simulink library "CurrentsLib"  (Simulink 7.7)
settings: Solver=ode45  SolverMode=SingleTasking  StartTime=0.0  StopTime=10.0  RelTol=1e-3
undefined symbols (not defined in the file or in its folder): A, B, diff1, EX, G, gX, PfAHP, PmAHP, PsAHP, Q0, S, T
libraries: CurrentsLib x75, WaveformsLib x11
(part 1 of 2)
settings Model: Creator=jpalma  LastModifiedBy=jpalma

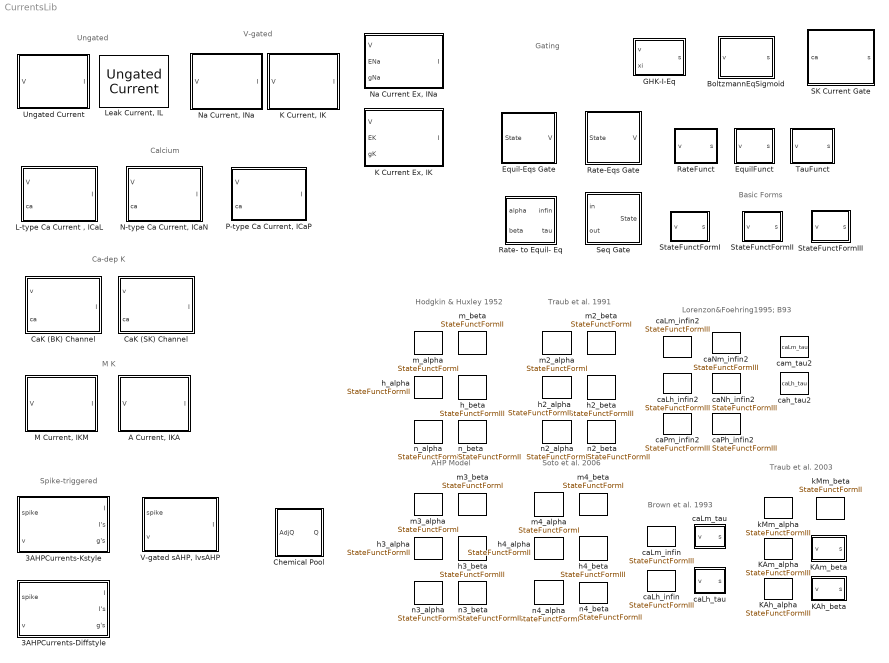
== system CurrentsLib ==
  note: Hodgkin & Huxley 1952
  note: Soto et al. 2006
  note: Basic Forms
  note: Traub et al. 1991
  note: AHP Model
  note: Gating
  note: V-gated
  note: Ungated
  note: Spike-triggered
  note: Brown et al. 1993
  note: Lorenzon&Foehring1995; B93
  note: Calcium
  note: Ca-dep K
  note: Traub et al. 2003
  note: M K
  3AHPCurrents-Diffstyle : Subsystem  mask{EfAHP=PfAHP(1), gfAHP=PfAHP(2), tauRfAHP=PfAHP(3), tauFfAHP=PfAHP(4), EmAHP=PmAHP(1), gmAHP=PmAHP(2), tauRmAHP=PmAHP(3), tauFmAHP=PmAHP(4), EsAHP=PsAHP(1), gsAHP=PsAHP(2), tauRsAHP=PsAHP(3), tauFsAHP=PsAHP(4)}
      mask prompts: EfAHP "Eq fAHP, EfAHP"; gfAHP "Conductance fAHP, gfAHP"; tauRfAHP "Rise Time fAHP"; tauFfAHP "Fall Time fAHP"; EmAHP "Eq mAHP, EmAHP"; gmAHP "Conductance mAHP, gmAHP"; tauRmAHP "Rise Time mAHP"; tauFmAHP "Fall Time mAHP"; EsAHP "Eq sAHP, EsAHP"; gsAHP "Conductance sAHP, gsAHP"; tauRsAHP "Rise Time sAHP"; tauFsAHP "Fall Time sAHP"
      mask help: Author: Jesse Palma
      mask Help: Author: Jesse Palma
      mask TabNameString: fAHP,fAHP,fAHP,fAHP,mAHP,mAHP,mAHP,mAHP,sAHP,sAHP,sAHP,sAHP
      mask Display: image(imread('../Libs/icons/ChannelV.jpg'),'center');
  3AHPCurrents-Kstyle : Subsystem  mask{EfAHP=PfAHP(1), gfAHP=PfAHP(2), tauRfAHP=PfAHP(3), tauFfAHP=PfAHP(4), EmAHP=PmAHP(1), gmAHP=PmAHP(2), tauRmAHP=PmAHP(3), tauFmAHP=PmAHP(4), EsAHP=PsAHP(1), gsAHP=PsAHP(2), tauRsAHP=PsAHP(3), tauFsAHP=PsAHP(4)}
      mask prompts: EfAHP "Eq fAHP, EfAHP"; gfAHP "Conductance fAHP, gfAHP"; tauRfAHP "Rise Time fAHP"; tauFfAHP "Fall Time fAHP"; EmAHP "Eq mAHP, EmAHP"; gmAHP "Conductance mAHP, gmAHP"; tauRmAHP "Rise Time mAHP"; tauFmAHP "Fall Time mAHP"; EsAHP "Eq sAHP, EsAHP"; gsAHP "Conductance sAHP, gsAHP"; tauRsAHP "Rise Time sAHP"; tauFsAHP "Fall Time sAHP"
      mask help: Author: Jesse Palma
      mask Help: Author: Jesse Palma
      mask TabNameString: fAHP,fAHP,fAHP,fAHP,mAHP,mAHP,mAHP,mAHP,sAHP,sAHP,sAHP,sAHP
      mask Display: image(imread('../Libs/icons/ChannelV.jpg'),'center');
  "A Current, IKA" : Subsystem  mask{EKA=-70, gKA=0.1, m_a=KAm_alpha, m_b=KAm_beta, h_a=KAh_alpha, h_b=KAh_beta}
      mask prompts: EKA "A Equilibrium, EKA (mV)"; gKA "A Conductance, gKA (mS/cm^2)"; m_a "Activation m Fwd Rate Eq, m_a"; m_b "Activation m Bckwd Rate Eq, m_b"; h_a "Inactivation h Fwd Rate Eq, h_a"; h_b "Inactivation h Bckwd Rate Eq, h_b"
      mask help:
      | Potassium A Current
      | IKA =  gKA m^4 h (EKA - V)
      |
      | (Traub et al. 2003)
      mask init:
      | set_param([gcb '/m Rate-Eqs Gate'], 'alphaF', m_a);
      | set_param([gcb '/m Rate-Eqs Gate'], 'betaF', m_b);
      | set_param([gcb '/h Rate-Eqs Gate'], 'alphaF', h_a);
      | set_param([gcb '/h Rate-Eqs Gate'], 'betaF', h_b);
      mask Help:
      | Potassium A Current
      | IKA =  gKA m^4 h (EKA - V)
      | 
      | (Traub et al. 2003)
      mask StyleString: edit,edit,popup(KAm_alpha),popup(KAm_beta),popup(KAh_alpha),popup(KAh_beta)
      mask TabNameString: Basic,Basic,Gating,Gating,Gating,Gating
      mask Display: image(imread('../Libs/icons/ChannelV.jpg'),'center');
  BoltzmannEqSigmoid : Subsystem  mask{v05=-20, k=1/5, g=4}
      mask prompts: v05 "Inflexion Point, v_0.5"; k "Slope factor, k"; g "Gain, g"
      mask help:
      | Boltzmann Equation as Sigmoid with Gain
      | [See (Dobois et al., 2009), doi:10.1016/j.pbiomolbio.2009.07.001]
      |
      |    s = g / (1 + exp((v_0.5-v)/k)
      |
      |    where k = zF/RT (slope factor)
      mask Help:
      | Boltzmann Equation as Sigmoid with Gain
      | [See (Dobois et al., 2009), doi:10.1016/j.pbiomolbio.2009.07.001]
      | 
      |    s = g / (1 + exp((v_0.5-v)/k))
      | 
      |    where k = zF/RT (Slope factor)
      mask Display: image(imread('../Libs/icons/SigmoidSF.jpg'),'center');
  CaK (BK) Channel : Subsystem  mask{EBK=-65, gBK=4.0}
      mask Display: image(imread('../Libs/icons/ChannelVC.jpg'),'center');
  CaK (SK) Channel : Subsystem  mask{ESK=-100, gSK=0.5}
      mask prompts: ESK "SK Equilibrium Potential, ESK"; gSK "SK Conductance, gSK"
      mask Display: image(imread('../Libs/icons/ChannelVC.jpg'),'center');
  Chemical Pool : Subsystem  mask{f=10/(69843), d=1/1000, a=1/200}
  Equil-Eqs Gate : Subsystem  mask{equilF=caLh_infin, tauF=caLh_tau}
      mask prompts: equilF "Equilbrium Eq (Steady State)"; tauF "Tau Eq (Time constant)"
      mask help: dF/dt = ( infty_F-F) / tau_F
      mask init:
      | set_param([gcb '/TauFunct'], 'BlockChoice', tauF);
      | set_param([gcb '/EquilFunct'], 'BlockChoice', equilF);
      mask Help: dF/dt = ( infty_F-F) / tau_F
      mask StyleString: popup(caLm_infin|caLh_infin|caLm_infin2|caLh_infin2|caNm_infin2|caNh_infin2|caPm_infin2|caPh_infin2),popup(caLm_tau|caLh_tau|cam_tau2|cah_tau2)
      mask Display: image(imread('../Libs/icons/EquilEq.jpg'),'center');
  EquilFunct : Subsystem  BlockChoice=caLh_infin
      settings: TemplateBlock=self  MemberBlocks=caLh_infin,caLh_infin2,caLm_infin,caLm_infin2,caNh_infin2,caNm_infin2,caPh_infin2,caPm_infin2
  GHK-I-Eq : Subsystem  mask{z=2, Xi=10*10^(-6), Xo=5, P=3.4*10^(-5)}
      mask prompts: z "Ion charge, z"; Xi "Internal concentration, Xi"; Xo "External concentration, Xo"; P "Permeability Scaling Factor, P"
      mask help:
      | GHK Current Equation
      |
      |    s = {PFz} kV (Xi-Xo exp (-kV))/(1 - exp(-kV))
      |
      |    where k = zF/RT
      |
      | {PFz} is a scaling factor, based on permeability
      |
      | z is the valence of ion
      | V is the transmembrane potential in volts
      | F is the Faraday constant, equal to 96,485 C·mol-1 or J·V-1·mol-1
      | R is the gas constant, equal to 8.314 J·K-1·mol-1
      | T is the absolute temperature, measured in kelvins (= degrees Celsius + 273.15)
      | Xi is the intracellular concentration of ion, measured in mol·m-3 or mmol·l-1
      | Xo is the extracellular concentration of ion, measured in mol·m-3
      mask Help:
      | GHK Current Equation
      | 
      |    s = {PFz} kV (Xi-Xo exp (-kV))/(1 - exp(-kV))
      | 
      |    where k = zF/RT
      | 
      | {PFz} is removed because it is scaling factor, which is performed outside this block
      | 
      | z is the valence of ion
      | V is the transmembrane potential in volts
      | F is the Faraday constant, equal to 96,485 C·mol-1 or J·V-1·mol-1
      | R is the gas constant, equal to 8.314 J·K-1·mol-1
      | T is the absolute temperature, measured in kelvins (= degrees Celsius + 273.15)
      | Xi is the intracellular concentration of ion, measured in mol·m-3 or mmol·l-1
      | Xo is the extracellular concentration of ion, measured in mol·m-3
  "K Current Ex, IK" : Subsystem  mask{n_a=n3_alpha, n_b=n3_beta}
      mask prompts: n_a "Activation n Fwd Rate Eq, n_a"; n_b "Activation n Bckwd Rate Eq, n_b"
      mask help:
      | Basic Potassium Current (Delayed Rectifier)
      |  IK =  gK n^4 (EK - V)
      |
      |  Model 1: Hodgkin & Huxley
      |  Model 2: Traub et al. 1991
      |  Model 3: AHP Model
      |           EK=-100 mV, gK = 16 mS/cm^2
      |  Model 4: Soto et al. 2006
      mask init:
      | set_param([gcb '/n Rate-Eqs Gate'], 'alphaF', n_a);
      | set_param([gcb '/n Rate-Eqs Gate'], 'betaF', n_b);
      mask Help:
      | Basic Potassium Current (Delayed Rectifier)
      |  IK =  gK n^4 (EK - V)
      | 
      |  Model 1: Hodgkin & Huxley
      |  Model 2: Traub et al. 1991
      |  Model 3: AHP Model
      |           EK=-100 mV, gK = 16 mS/cm^2
      |  Model 4: Soto et al. 2006
      mask StyleString: popup(n_alpha|n2_alpha|n3_alpha|n4_alpha),popup(n_beta|n2_beta|n3_beta|n4_beta)
      mask TabNameString: Gating,Gating
      mask Display: image(imread('../Libs/icons/ChannelV.jpg'),'center');
  "K Current, IK" : Subsystem  mask{EK=-100, gK=16, n_a=n3_alpha, n_b=n3_beta}
      mask prompts: EK "Potassium Equilibrium, EK (mV)"; gK "Potassium Conductance, gK (mS/cm^2)"; n_a "Activation n Fwd Rate Eq, n_a"; n_b "Activation n Bckwd Rate Eq, n_b"
      mask help:
      | Basic Potassium Current (Delayed Rectifier)
      |  IK =  gK n^4 (EK - V)
      |
      |  Model 1: Hodgkin & Huxley
      |  Model 2: Traub et al. 1991
      |  Model 3: AHP Model
      |           EK=-100 mV, gK = 16 mS/cm^2
      |  Model 4: Soto et al. 2006
      mask init:
      | set_param([gcb '/n Rate-Eqs Gate'], 'alphaF', n_a);
      | set_param([gcb '/n Rate-Eqs Gate'], 'betaF', n_b);
      mask Help:
      | Basic Potassium Current (Delayed Rectifier)
      |  IK =  gK n^4 (EK - V)
      | 
      |  Model 1: Hodgkin & Huxley
      |  Model 2: Traub et al. 1991
      |  Model 3: AHP Model
      |           EK=-100 mV, gK = 16 mS/cm^2
      |  Model 4: Soto et al. 2006
      mask StyleString: edit,edit,popup(n_alpha|n2_alpha|n3_alpha|n4_alpha),popup(n_beta|n2_beta|n3_beta|n4_beta)
      mask TabNameString: Basic,Basic,Gating,Gating
      mask Display: image(imread('../Libs/icons/ChannelV.jpg'),'center');
  KAh_alpha : CurrentsLib/StateFunctFormIII  SystemSampleTime=-1  T=-85  S=-1/16  B=1  G=1/8
  KAh_beta : Subsystem
      mask Description: 1.2
      mask Help: 1.2
  KAm_alpha : CurrentsLib/StateFunctFormIII  SystemSampleTime=-1  T=-28  S=1/22.5  B=1  G=1/8
  KAm_beta : Subsystem
  "L-type Ca Current , ICaL" : Subsystem  mask{ECaL=130, gCaL=0.1, m_e=caLm_infin2, m_t=cam_tau2, h_e=caLh_infin2, h_t=cah_tau2}
      mask prompts: ECaL "Sodium Equilibrium, ECaL (mV)"; gCaL "Sodium Conductance, gCaL (mS/cm^2)"; m_e "Activation m Equil Eq, m_e"; m_t "Activation m Tau Eq, m_t"; h_e "Inactivation h Equil Eq, h_e"; h_t "Inactivation h Tau Eq, h_t"
      mask help:
      | L-type Calcium Current
      | ICaL =  gCaL m^2 h (ECaL - V)
      |
      | Based on (Brown et al. 1993)
      mask init:
      | set_param([gcb '/m Equil-Eqs Gate'], 'equilF', m_e);
      | set_param([gcb '/m Equil-Eqs Gate'], 'tauF', m_t);
      | set_param([gcb '/h Equil-Eqs Gate'], 'equilF', h_e);
      | set_param([gcb '/h Equil-Eqs Gate'], 'tauF', h_t);
      mask Help:
      | L-type Calcium Current
      | ICaL =  gCaL m^2 h (ECaL - V)
      | 
      | Based on (Brown et al. 1993)
      mask StyleString: edit,edit,popup(caLm_infin|caLm_infin2),popup(caLm_tau|cam_tau2),popup(caLh_infin|caLh_infin2),popup(caLh_tau|cah_tau2)
      mask TabNameString: Basic,Basic,Gating,Gating,Gating,Gating
      mask Display: image(imread('../Libs/icons/ChannelV.jpg'),'center');
  "Leak Current, IL" : CurrentsLib/Ungated Current  SystemSampleTime=-1  EX=-65  gX=0.1
  "M Current, IKM" : Subsystem  mask{EK=-100, gK=0.1, m_a=kMm_alpha, m_b=kMm_beta}
      mask prompts: EK "Potassium Equilibrium, EK (mV)"; gK "Potassium Conductance, gK (mS/cm^2)"; m_a "Activation m Fwd Rate Eq, m_a"; m_b "Activation m Bckwd Rate Eq, m_b"
      mask help: Potassium M Current (Traub et al. 2003)
      mask init:
      | set_param([gcb '/m Rate-Eqs Gate'], 'alphaF', m_a);
      | set_param([gcb '/m Rate-Eqs Gate'], 'betaF', m_b);
      mask Help: Potassium M Current (Traub et al. 2003)
      mask StyleString: edit,edit,popup(kMm_alpha),popup(kMm_beta)
      mask TabNameString: Basic,Basic,Gating,Gating
      mask Display: image(imread('../Libs/icons/ChannelV.jpg'),'center');
  "N-type Ca Current, ICaN" : Subsystem  mask{ECaN=130, gCaN=0.1, m_e=caNm_infin2, m_t=cam_tau2, h_e=caNh_infin2, h_t=cah_tau2}
      mask prompts: ECaN "Sodium Equilibrium, ECaN (mV)"; gCaN "Sodium Conductance, gCaN (mS/cm^2)"; m_e "Activation m Equil Eq, m_e"; m_t "Activation m Tau Eq, m_t"; h_e "Inactivation h Equil Eq, h_e"; h_t "Inactivation h Tau Eq, h_t"
      mask help:
      | N-type Calcium Current
      | ICaN =  gCaN m h (ECaN - V)
      mask init: same as CurrentsLib/L-type Ca Current , ICaL
      mask Help:
      | N-type Calcium Current
      | ICaN =  gCaN m h (ECaN - V)
      mask StyleString: edit,edit,popup(caNm_infin|caNm_infin2),popup(caNm_tau|cam_tau2),popup(caNh_infin|caNh_infin2),popup(caNh_tau|cah_tau2)
      mask TabNameString: Basic,Basic,Gating,Gating,Gating,Gating
      mask Display: image(imread('../Libs/icons/ChannelV.jpg'),'center');
  "Na Current Ex, INa" : Subsystem  mask{m_a=m3_alpha, m_b=m3_beta, h_a=h3_alpha, h_b=h3_beta}
      mask prompts: m_a "Activation m Fwd Rate Eq, m_a"; m_b "Activation m Bckwd Rate Eq, m_b"; h_a "Inactivation h Fwd Rate Eq, h_a"; h_b "Inactivation h Bckwd Rate Eq, h_b"
      mask help:
      | Basic Sodium Current
      | INa =  gNa m^3 h (ENa - V)
      |
      |  Model 1: Hodgkin & Huxley
      |  Model 2: Traub et al. 1991
      |  Model 3: AHP Model
      |           ENa=50 mV, gNa = 45 mS/cm^2
      |  Model 4: Soto et al. 2006
      mask init: same as CurrentsLib/A Current, IKA
      mask Help:
      | Basic Sodium Current
      | INa =  gNa m^3 h (ENa - V)
      | 
      |  Model 1: Hodgkin & Huxley
      |  Model 2: Traub et al. 1991
      |  Model 3: AHP Model
      |           ENa=50 mV, gNa = 45 mS/cm^2
      |  Model 4: Soto et al. 2006
      mask StyleString: popup(m_alpha|m2_alpha|m3_alpha|m4_alpha),popup(m_beta|m2_beta|m3_beta|m4_beta),popup(h_alpha|h2_alpha|h3_alpha|h4_alpha),popup(h_beta|h2_beta|h3_beta|h4_beta)
      mask TabNameString: Gating,Gating,Gating,Gating
      mask Display: image(imread('../Libs/icons/ChannelV.jpg'),'center');
  "Na Current, INa" : Subsystem  mask{ENa=50, gNa=45, m_a=m3_alpha, m_b=m3_beta, h_a=h3_alpha, h_b=h3_beta}
      mask prompts: ENa "Sodium Equilibrium, ENa (mV)"; gNa "Sodium Conductance, gNa (mS/cm^2)"; m_a "Activation m Fwd Rate Eq, m_a"; m_b "Activation m Bckwd Rate Eq, m_b"; h_a "Inactivation h Fwd Rate Eq, h_a"; h_b "Inactivation h Bckwd Rate Eq, h_b"
      mask help:
      | Basic Sodium Current
      | INa =  gNa m^3 h (ENa - V)
      |
      |  Model 1: Hodgkin & Huxley
      |  Model 2: Traub et al. 1991
      |  Model 3: AHP Model
      |           ENa=50 mV, gNa = 45 mS/cm^2
      |  Model 4: Soto et al. 2006
      mask init: same as CurrentsLib/A Current, IKA
      mask Help:
      | Basic Sodium Current
      | INa =  gNa m^3 h (ENa - V)
      | 
      |  Model 1: Hodgkin & Huxley
      |  Model 2: Traub et al. 1991
      |  Model 3: AHP Model
      |           ENa=50 mV, gNa = 45 mS/cm^2
      |  Model 4: Soto et al. 2006
      mask StyleString: edit,edit,popup(m_alpha|m2_alpha|m3_alpha|m4_alpha),popup(m_beta|m2_beta|m3_beta|m4_beta),popup(h_alpha|h2_alpha|h3_alpha|h4_alpha),popup(h_beta|h2_beta|h3_beta|h4_beta)
      mask TabNameString: Basic,Basic,Gating,Gating,Gating,Gating
      mask Display: image(imread('../Libs/icons/ChannelV.jpg'),'center');
  "P-type Ca Current, ICaP" : Subsystem  mask{ECaP=130, gCaP=0.1, m_e=caPm_infin2, m_t=cam_tau2, h_e=caPh_infin2, h_t=cah_tau2}
      mask prompts: ECaP "Sodium Equilibrium, ECaP (mV)"; gCaP "Sodium Conductance, gCaP (mS/cm^2)"; m_e "Activation m Equil Eq, m_e"; m_t "Activation m Tau Eq, m_t"; h_e "Inactivation h Equil Eq, h_e"; h_t "Inactivation h Tau Eq, h_t"
      mask help:
      | P-type Calcium Current
      | ICaP =  gCaP m h (ECaP - V)
      mask init: same as CurrentsLib/L-type Ca Current , ICaL
      mask Help:
      | P-type Calcium Current
      | ICaP =  gCaP m h (ECaP - V)
      mask StyleString: edit,edit,popup(caPm_infin|caPm_infin2),popup(caPm_tau|cam_tau2),popup(caPh_infin|caPh_infin2),popup(caPh_tau|cah_tau2)
      mask TabNameString: Basic,Basic,Gating,Gating,Gating,Gating
      mask Display: image(imread('../Libs/icons/ChannelV.jpg'),'center');
  Rate- to Equil- Eq : Subsystem
      mask Description: Converts Rate Eqs to Equil Eqs
      mask Help: Converts Rate Eqs to Equil Eqs
      mask Display: image(imread('../Libs/icons/Rate2Equil.jpg'),'center');
  Rate-Eqs Gate : Subsystem  mask{alphaF=m3_alpha, betaF=m3_beta}
      mask prompts: alphaF "Forward Rate Eq"; betaF "Backward Rate Eq"
      mask help: dF/dt = alpha_F(1-F) - beta_F*F
      mask init:
      | set_param([gcb '/RateFunctA'], 'BlockChoice', alphaF);
      | set_param([gcb '/RateFunctB'], 'BlockChoice', betaF);
      mask Help: dF/dt =  alpha_F(1-F) - beta_F*F
      mask StyleString: popup(m_alpha|h_alpha|n_alpha|m2_alpha|h2_alpha|n2_alpha|m3_alpha|h3_alpha|n3_alpha|m4_alpha|h4_alpha|n4_alpha|kMm_alpha|KAm_alpha|KAh_alpha),popup(m_beta|h_beta|n_beta|m2_beta|h2_beta|n2_beta|m3_beta|h3_beta|n3_beta|m4_beta|h4_beta|n4_beta|kMm_beta|KAm_beta|KAh_beta)
      mask Display: image(imread('../Libs/icons/RateEq.jpg'),'center');
  RateFunct : Subsystem  BlockChoice=m_alpha
      settings: TemplateBlock=self  MemberBlocks=KAh_alpha,KAh_beta,KAm_alpha,KAm_beta,caLh_infin,caLh_infin2,caLh_tau,caLm_infin,caLm_infin2,caLm_tau,caNh_infin2,caNm_infin2,caPh_infin2,caPm_infin2,cah_tau2,cam_tau2,h2_alpha,h2_beta,h3_alpha,h3_beta,h4_alpha,h4_beta,h_alpha,h_beta,kMm_alpha,kMm_beta,m2_alpha,m2_beta,m3_alpha,m3_beta,m4_alpha,m4_beta,m_alpha,m_beta,n2_alpha,n2_beta,n3_alpha,n3_beta,n4_alpha,n4_beta,n_alpha,n_beta
  SK Current Gate : Subsystem
      mask Description: Based on (Hirschberg et al, 1998)
      mask Help: Based on (Hirschberg et al, 1998)
      mask Display: image(imread('../Libs/icons/SKGate.jpg'),'center');
  Seq Gate : Subsystem  mask{S0=0}
      mask prompts: S0 "Initial State"
      mask help: dF/dt = in - out*F
      mask Help: dF/dt =  in - out*F
      mask Display: image(imread('../Libs/icons/RateEq.jpg'),'center');
  StateFunctFormI : Subsystem  mask{T=-47, S=1/4, M=-1, B=1, G=0.32}
      mask prompts: T "Turnpoint, T"; S "Slope, S"; M "MidGain, M"; B "MidBias, B"; G "Final Gain, G"
      mask help:
      | s = G (T-v) / (- M exp(S(T-v)) - B)
      |
      | OR
      |
      | s = G (v-T) / (B + M exp(-S(v-T)))
      mask Help:
      | s = G (T-v) / (- M exp(S(T-v)) - B)
      | 
      | OR
      | 
      | s = G (v-T) / (B + M exp(-S(v-T)))
  StateFunctFormII : Subsystem  mask{T=-43, S=1/18, G=0.128}
      mask prompts: T "Turnpoint, T"; S "Slope, S"; G "Final Gain, G"
      mask help:
      | s = G exp( S(T-v))
      |
      | OR
      |
      | s = G exp( -S(v-T))
      mask Help:
      | s = G exp( S(T-v))
      | 
      | OR
      | 
      | s = G exp( -S(v-T))
  StateFunctFormIII : Subsystem  mask{T=-20, S=1/5, B=1, G=4}
      mask prompts: T "Turnpoint, T"; S "Slope, S"; B "Mid Bias, B"; G "Final Gain, G"
      mask help:
      | s = G / (exp(S(T-v)) + B)
      |
      | OR
      |
      | s = G / (exp(-S(v-T)) + B)
      mask Help:
      | s = G / (exp(S(T-v)) + B)
      | 
      | OR
      | 
      | s = G / (exp(-S(v-T)) + B)
  TauFunct : Subsystem  BlockChoice=caLh_tau
      settings: TemplateBlock=self  MemberBlocks=caLh_tau,caLm_tau,cah_tau2,cam_tau2
  Ungated Current : Subsystem  mask{EX=EX, gX=gX}
      mask prompts: EX "Equilibrium, EX (mV)"; gX "Conductance, gX (mS/cm^2)"
      mask help:
      | A simple ungated current follows Ohm's Law.
      | IX =  gX (EX - V)
      mask Help:
      | A simple ungated current follows Ohm's Law.
      | IX =  gX (EX - V)
      mask Display: image(imread('../Libs/icons/Channel.JPG'),'center');
  "V-gated sAHP, IvsAHP" : Subsystem  mask{EvsAHP=-100, gvsAHP=0.1, RvsAHP=225, FvsAHP=2400}
      mask prompts: EvsAHP "V sAHP Equilbrium"; gvsAHP "V sAHP Conductance"; RvsAHP "Rise Time"; FvsAHP "Fall Time"
      mask Display: image(imread('../Libs/icons/ChannelV.jpg'),'center');
  caLh_infin : CurrentsLib/StateFunctFormIII  SystemSampleTime=-1  T=-12.6  S=1/18.9  B=1  G=1
  caLh_infin2 : CurrentsLib/StateFunctFormIII  SystemSampleTime=-1  T=-20  S=-1/5  B=1  G=1
  caLh_tau : Subsystem
      mask Description: 420
      mask Help: 420
  caLm_infin : CurrentsLib/StateFunctFormIII  SystemSampleTime=-1  T=-24.6  S=1/11.3  B=1  G=1
  caLm_infin2 : CurrentsLib/StateFunctFormIII  SystemSampleTime=-1  T=-20  S=1/5  B=1  G=1
  caLm_tau : Subsystem
  caNh_infin2 : CurrentsLib/StateFunctFormIII  SystemSampleTime=-1  T=-20  S=-1/5  B=1  G=1
  caNm_infin2 : CurrentsLib/StateFunctFormIII  SystemSampleTime=-1  T=-20  S=1/5  B=1  G=1
  caPh_infin2 : CurrentsLib/StateFunctFormIII  SystemSampleTime=-1  T=-18  S=-1/5.5  B=1  G=1
  caPm_infin2 : CurrentsLib/StateFunctFormIII  SystemSampleTime=-1  T=-18  S=1/5.5  B=1  G=1
  cah_tau2 : CurrentsLib/caLh_tau  SystemSampleTime=-1
  cam_tau2 : CurrentsLib/caLm_tau  SystemSampleTime=-1
  h2_alpha : CurrentsLib/StateFunctFormII  SystemSampleTime=-1  T=-43  S=1/18  G=0.128
  h2_beta : CurrentsLib/StateFunctFormIII  SystemSampleTime=-1  T=-20  S=0.2  B=1  G=4
  h3_alpha : CurrentsLib/StateFunctFormII  SystemSampleTime=-1  T=-43  S=1/18  G=0.128
  h3_beta : CurrentsLib/StateFunctFormIII  SystemSampleTime=-1  T=-20  S=0.2  B=1  G=4
  h4_alpha : CurrentsLib/StateFunctFormII  SystemSampleTime=-1  T=-50  S=1/18  G=0.128
  h4_beta : CurrentsLib/StateFunctFormIII  SystemSampleTime=-1  T=-27  S=1/5  B=1  G=4
  h_alpha : CurrentsLib/StateFunctFormII  SystemSampleTime=-1  T=-60  S=1/20  G=0.07
  h_beta : CurrentsLib/StateFunctFormIII  SystemSampleTime=-1  T=-30  S=1/10  B=1  G=1
  kMm_alpha : CurrentsLib/StateFunctFormIII  SystemSampleTime=-1  T=-25  S=1/5  B=1  G=0.002
  kMm_beta : CurrentsLib/StateFunctFormII  SystemSampleTime=-1  T=-45  S=1/6  G=0.001
  m2_alpha : CurrentsLib/StateFunctFormI  SystemSampleTime=-1  T=-46.9  S=0.25  M=-1  B=1  G=0.32
  m2_beta : CurrentsLib/StateFunctFormI  SystemSampleTime=-1  T=-19.9  S=-0.2  M=1  B=-1  G=0.28
  m3_alpha : CurrentsLib/StateFunctFormI  SystemSampleTime=-1  T=-47  S=0.25  M=-1  B=1  G=0.32
  m3_beta : CurrentsLib/StateFunctFormI  SystemSampleTime=-1  T=-20  S=-0.2  M=1  B=-1  G=0.28
  m4_alpha : CurrentsLib/StateFunctFormI  SystemSampleTime=-1  T=-50  S=1/4  M=-1  B=1  G=0.32
  m4_beta : CurrentsLib/StateFunctFormI  SystemSampleTime=-1  T=-27  S=-1/5  M=1  B=-1  G=0.28
  m_alpha : CurrentsLib/StateFunctFormI  SystemSampleTime=-1  T=-35  S=1/10  M=-1  B=1  G=0.1
  m_beta : CurrentsLib/StateFunctFormII  SystemSampleTime=-1  T=-60  S=1/18  G=4
  n2_alpha : CurrentsLib/StateFunctFormI  SystemSampleTime=-1  T=-24.9  S=0.2  M=-1  B=1  G=0.016
  n2_beta : CurrentsLib/StateFunctFormII  SystemSampleTime=-1  T=-40  S=1/40  G=0.25
  n3_alpha : CurrentsLib/StateFunctFormI  SystemSampleTime=-1  T=-45  S=0.2  M=-1  B=1  G=0.012
  n3_beta : CurrentsLib/StateFunctFormII  SystemSampleTime=-1  T=-50  S=1/40  G=0.5
  n4_alpha : CurrentsLib/StateFunctFormI  SystemSampleTime=-1  T=-52  S=1/5  M=-1  B=1  G=0.032
  n4_beta : CurrentsLib/StateFunctFormII  SystemSampleTime=-1  T=-57  S=1/40  G=0.5
  n_alpha : CurrentsLib/StateFunctFormI  SystemSampleTime=-1  T=-50  S=1/10  M=-1  B=1  G=0.01
  n_beta : CurrentsLib/StateFunctFormII  SystemSampleTime=-1  T=-60  S=1/80  G=0.125

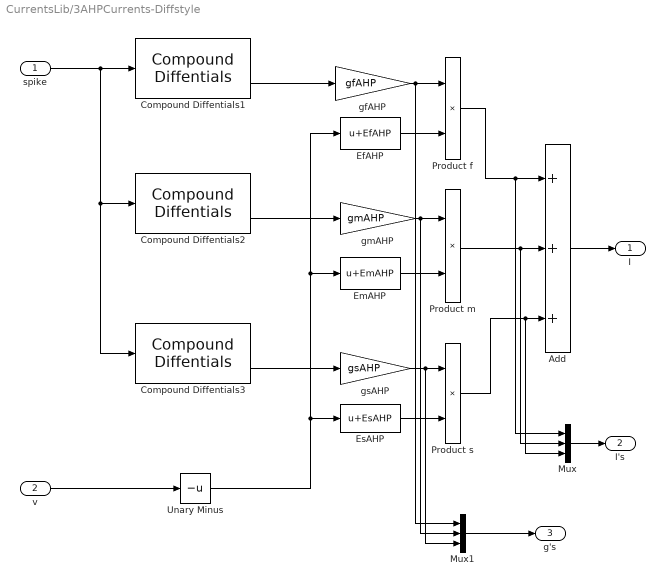
== system CurrentsLib/3AHPCurrents-Diffstyle ==
  spike : Inport
  v : Inport  Port=2
  Add : Sum  Inputs=+++
  Compound Diffentials1 : WaveformsLib/Compound Diffentials  SystemSampleTime=-1  tauRise=tauRfAHP  tauFall=tauFfAHP  squareWaveWidth=tauRfAHP  squareWaveHeight=1/tauRfAHP  interGain=2/tauRfAHP  finalGain=(tauFfAHP+tauRfAHP)/(1*tauFfAHP)
  Compound Diffentials2 : WaveformsLib/Compound Diffentials  SystemSampleTime=-1  tauRise=tauRmAHP  tauFall=tauFmAHP  squareWaveWidth=tauRmAHP  squareWaveHeight=1/tauRmAHP  interGain=2/tauRmAHP  finalGain=(tauFmAHP+tauRmAHP)/(1*tauFmAHP)
  Compound Diffentials3 : WaveformsLib/Compound Diffentials  SystemSampleTime=-1  tauRise=tauRsAHP  tauFall=tauFsAHP  squareWaveWidth=tauRsAHP  squareWaveHeight=1/tauRsAHP  interGain=2/tauRsAHP  finalGain=(tauFsAHP+tauRsAHP)/(1*tauFsAHP)
  EfAHP : Bias  Bias=EfAHP
  EmAHP : Bias  Bias=EmAHP
  EsAHP : Bias  Bias=EsAHP
  Mux : Mux  Inputs=3
  Mux1 : Mux  Inputs=3
  Product f : Product  RndMeth=Zero
  Product m : Product  RndMeth=Zero
  Product s : Product  RndMeth=Zero
  Unary Minus : UnaryMinus
  gfAHP : Gain  Gain=gfAHP
  gmAHP : Gain  Gain=gmAHP
  gsAHP : Gain  Gain=gsAHP
  I : Outport
  I's : Outport  Port=2
  g's : Outport  Port=3
  wires:
  Mux1/1 -> g's/1
  Mux/1 -> I's/1
  Unary Minus/1 -> EsAHP/1, EmAHP/1, EfAHP/1
  Product s/1 -> Mux/3, Add/3
  Product m/1 -> Mux/2, Add/2
  Product f/1 -> Mux/1, Add/1
  v/1 -> Unary Minus/1
  spike/1 -> Compound Diffentials2/1, Compound Diffentials3/1, Compound Diffentials1/1
  Compound Diffentials3/2 -> gsAHP/1
  EsAHP/1 -> Product s/2
  gsAHP/1 -> Mux1/3, Product s/1
  Compound Diffentials2/2 -> gmAHP/1
  EmAHP/1 -> Product m/2
  gmAHP/1 -> Mux1/2, Product m/1
  Compound Diffentials1/2 -> gfAHP/1
  EfAHP/1 -> Product f/2
  gfAHP/1 -> Mux1/1, Product f/1
  Add/1 -> I/1

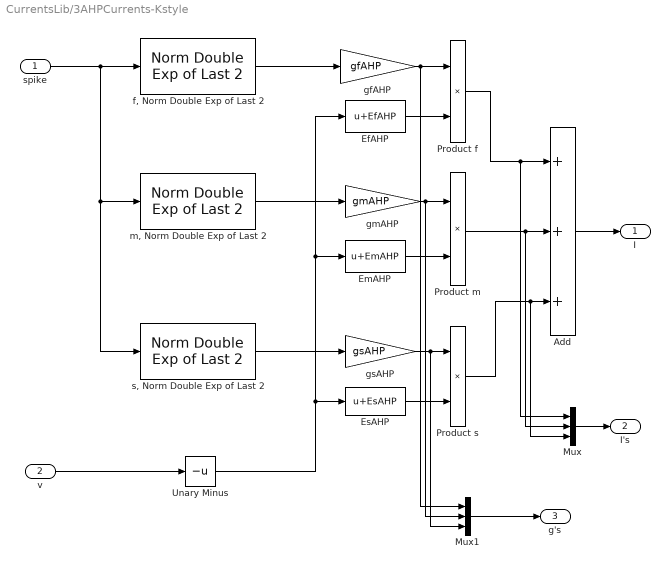
== system CurrentsLib/3AHPCurrents-Kstyle ==
  spike : Inport
  v : Inport  Port=2
  Add : Sum  Inputs=+++
  EfAHP : Bias  Bias=EfAHP
  EmAHP : Bias  Bias=EmAHP
  EsAHP : Bias  Bias=EsAHP
  Mux : Mux  Inputs=3
  Mux1 : Mux  Inputs=3
  Product f : Product  RndMeth=Zero
  Product m : Product  RndMeth=Zero
  Product s : Product  RndMeth=Zero
  Unary Minus : UnaryMinus
  "f, Norm Double Exp of Last 2" : WaveformsLib/Norm Double Exp of Last 2  SystemSampleTime=-1  tauRise=tauRfAHP  tauFall=tauFfAHP
  gfAHP : Gain  Gain=gfAHP
  gmAHP : Gain  Gain=gmAHP
  gsAHP : Gain  Gain=gsAHP
  "m, Norm Double Exp of Last 2" : WaveformsLib/Norm Double Exp of Last 2  SystemSampleTime=-1  tauRise=tauRmAHP  tauFall=tauFmAHP
  "s, Norm Double Exp of Last 2" : WaveformsLib/Norm Double Exp of Last 2  SystemSampleTime=-1  tauRise=tauRsAHP  tauFall=tauFsAHP
  I : Outport
  I's : Outport  Port=2
  g's : Outport  Port=3
  wires:
  Add/1 -> I/1
  gfAHP/1 -> Product f/1, Mux1/1
  EfAHP/1 -> Product f/2
  "f, Norm Double Exp of Last 2"/1 -> gfAHP/1
  gmAHP/1 -> Product m/1, Mux1/2
  EmAHP/1 -> Product m/2
  "m, Norm Double Exp of Last 2"/1 -> gmAHP/1
  gsAHP/1 -> Product s/1, Mux1/3
  EsAHP/1 -> Product s/2
  "s, Norm Double Exp of Last 2"/1 -> gsAHP/1
  spike/1 -> "m, Norm Double Exp of Last 2"/1, "s, Norm Double Exp of Last 2"/1, "f, Norm Double Exp of Last 2"/1
  v/1 -> Unary Minus/1
  Product f/1 -> Add/1, Mux/1
  Product m/1 -> Add/2, Mux/2
  Product s/1 -> Add/3, Mux/3
  Unary Minus/1 -> EsAHP/1, EfAHP/1, EmAHP/1
  Mux/1 -> I's/1
  Mux1/1 -> g's/1

== system CurrentsLib/A Current, IKA ==
  note: I_{KA} = g_{KA} m^4 h (E_{KA} - V)
  V : Inport
  " 3" : Constant  Value=4
  4th : Math  Operator=pow  SaturateOnIntegerOverflow=on
  Product : Product  Inputs=3  RndMeth=Zero
  "Ungated Current, gKA (EKA - V)" : CurrentsLib/Ungated Current  SystemSampleTime=-1  EX=EKA  gX=gKA
  h Rate-Eqs Gate : CurrentsLib/Rate-Eqs Gate  SystemSampleTime=-1  alphaF=KAh_alpha  betaF=KAh_beta
  m Rate-Eqs Gate : CurrentsLib/Rate-Eqs Gate  SystemSampleTime=-1  alphaF=KAm_alpha  betaF=KAm_beta
  I : Outport
  wires:
  Product/1 -> I/1
  "Ungated Current, gKA (EKA - V)"/1 -> Product/3
  V/1 -> "Ungated Current, gKA (EKA - V)"/1, h Rate-Eqs Gate/1, m Rate-Eqs Gate/1
  " 3"/1 -> 4th/2
  m Rate-Eqs Gate/1 -> 4th/1
  4th/1 -> Product/1
  h Rate-Eqs Gate/1 -> Product/2

== system CurrentsLib/BoltzmannEqSigmoid ==
  note: s = G ./ (exp( -S*(-T+v)) + B)
  v : Inport
  Gain : Gain  Gain=G
  Slope : Gain  Gain=-S
  Turn : Bias  Bias=-T
  Turn1 : Bias  Bias=B
  exp : Math  SaturateOnIntegerOverflow=on
  recip : Math  Operator=reciprocal  SaturateOnIntegerOverflow=on
  s : Outport
  wires:
  recip/1 -> Gain/1
  Turn1/1 -> recip/1
  Turn/1 -> Slope/1
  Slope/1 -> exp/1
  v/1 -> Turn/1
  Gain/1 -> s/1
  exp/1 -> Turn1/1

== system CurrentsLib/CaK (BK) Channel ==
  v : Inport
  ca : Inport  Port=2
  Product1 : Product  RndMeth=Zero
  Ungated Current : CurrentsLib/Ungated Current  SystemSampleTime=-1  EX=EBK  gX=gBK
  p-gate : Subsystem
  I : Outport
  wires:
  ca/1 -> p-gate/2(ca)
  p-gate/1(p) -> Product1/1
  Product1/1 -> I/1
  Ungated Current/1 -> Product1/2
  v/1 -> p-gate/1(v), Ungated Current/1

== system CurrentsLib/CaK (SK) Channel ==
  v : Inport
  ca : Inport  Port=2
  Product : Product  RndMeth=Zero
  SK Equil : CurrentsLib/Ungated Current  SystemSampleTime=-1  EX=ESK  gX=gSK
  SK Gate : CurrentsLib/SK Current Gate  SystemSampleTime=-1
  I : Outport
  wires:
  Product/1 -> I/1
  v/1 -> SK Equil/1
  ca/1 -> SK Gate/1
  SK Equil/1 -> Product/1
  SK Gate/1 -> Product/2

== system CurrentsLib/Chemical Pool ==
  AdjQ : Inport
  Leaky Integrator : WaveformsLib/Leaky Integrator  SystemSampleTime=-1  X0=Q0  A=A
  QDiff : Sum  Inputs=+-
  d : Gain  Gain=diff1
  Q : Outport
  wires:
  d/1 -> Leaky Integrator/1
  QDiff/1 -> d/1
  AdjQ/1 -> QDiff/1
  Leaky Integrator/1 -> Q/1, QDiff/2

== system CurrentsLib/Equil-Eqs Gate ==
  note: dF/dt = ( \infty _F-F) / \tau_F
  V : Inport
  Add1 : Sum  Inputs=-+
  Divide : Product  Inputs=*/
  EquilFunct : Subsystem  BlockChoice=caLh_infin
      settings: AttributesFormatString=%<BlockChoice>  TemplateBlock=CurrentsLib/EquilFunct  MemberBlocks=caLh_infin,caLh_infin2,caLm_infin,caLm_infin2,caNh_infin2,caNm_infin2,caPh_infin2,caPm_infin2
  Integrator : Integrator
  TauFunct : Subsystem  BlockChoice=caLh_tau
      settings: AttributesFormatString=%<BlockChoice>  TemplateBlock=CurrentsLib/TauFunct  MemberBlocks=caLh_tau,caLm_tau,cah_tau2,cam_tau2
  State : Outport
  wires:
  Integrator/1 -> Add1/1, State/1
  Add1/1 -> Divide/1
  Divide/1 -> Integrator/1
  TauFunct/1(s) -> Divide/2
  EquilFunct/1(s) -> Add1/2
  V/1 -> TauFunct/1(v), EquilFunct/1(v)

== system CurrentsLib/EquilFunct ==
  v : Inport
  caLh_infin : CurrentsLib/StateFunctFormIII  SystemSampleTime=-1  T=-12.6  S=1/18.9  B=1  G=1
  s : Outport
  wires:
  v/1 -> caLh_infin/1
  caLh_infin/1 -> s/1

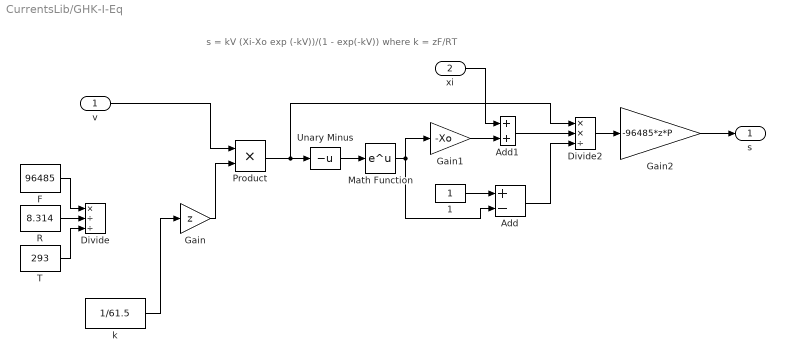
== system CurrentsLib/GHK-I-Eq ==
  note: s = kV (Xi-Xo exp (-kV))/(1 - exp(-kV))
      |
      |    where k = zF/RT
  v : Inport
  xi : Inport  Port=2
  1 : Constant
  Add : Sum  Inputs=+-
  Add1 : Sum
  Divide : Product  Inputs=*//
  Divide2 : Product  Inputs=**/
  F : Constant  Value=96485
  Gain : Gain  Gain=z
  Gain1 : Gain  Gain=-Xo
  Gain2 : Gain  Gain=-96485*z*P
  Math Function : Math  SaturateOnIntegerOverflow=on
  Product : Product  RndMeth=Zero
  R : Constant  Value=8.314
  T : Constant  Value=293
  Unary Minus : UnaryMinus
  k : Constant  Value=1/61.5
  s : Outport
  wires:
  k/1 -> Gain/1
  Divide2/1 -> Gain2/1
  v/1 -> Product/1
  F/1 -> Divide/1
  R/1 -> Divide/2
  T/1 -> Divide/3
  Gain/1 -> Product/2
  Product/1 -> Unary Minus/1, Divide2/1
  Unary Minus/1 -> Math Function/1
  Math Function/1 -> Add/2, Gain1/1
  Gain1/1 -> Add1/2
  Add1/1 -> Divide2/2
  Add/1 -> Divide2/3
  1/1 -> Add/1
  Gain2/1 -> s/1
  xi/1 -> Add1/1

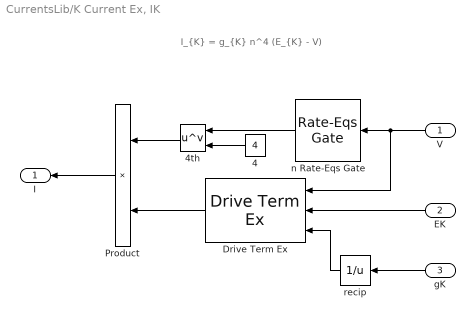
== system CurrentsLib/K Current Ex, IK ==
  note: I_{K} = g_{K} n^4 (E_{K} - V)
  V : Inport
  EK : Inport  Port=2
  gK : Inport  Port=3
  " 4" : Constant  Value=4
  4th : Math  Operator=pow  SaturateOnIntegerOverflow=on
  Drive Term Ex : WaveformsLib/Drive Term Ex  SystemSampleTime=-1
  Product : Product  RndMeth=Zero
  n Rate-Eqs Gate : CurrentsLib/Rate-Eqs Gate  SystemSampleTime=-1  alphaF=n3_alpha  betaF=n3_beta
  recip : Math  Operator=reciprocal  SaturateOnIntegerOverflow=on
  I : Outport
  wires:
  Drive Term Ex/1 -> Product/2
  Product/1 -> I/1
  4th/1 -> Product/1
  n Rate-Eqs Gate/1 -> 4th/1
  " 4"/1 -> 4th/2
  V/1 -> n Rate-Eqs Gate/1, Drive Term Ex/1
  EK/1 -> Drive Term Ex/2
  gK/1 -> recip/1
  recip/1 -> Drive Term Ex/3

== system CurrentsLib/K Current, IK ==
  note: I_{K} = g_{K} n^4 (E_{K} - V)
  V : Inport
  " 4" : Constant  Value=4
  4th : Math  Operator=pow  SaturateOnIntegerOverflow=on
  Product : Product  RndMeth=Zero
  "Ungated Current, gK (EK - V)" : CurrentsLib/Ungated Current  SystemSampleTime=-1  EX=EK  gX=gK
  n Rate-Eqs Gate : CurrentsLib/Rate-Eqs Gate  SystemSampleTime=-1  alphaF=n3_alpha  betaF=n3_beta
  I : Outport
  wires:
  V/1 -> n Rate-Eqs Gate/1, "Ungated Current, gK (EK - V)"/1
  " 4"/1 -> 4th/2
  n Rate-Eqs Gate/1 -> 4th/1
  4th/1 -> Product/1
  Product/1 -> I/1
  "Ungated Current, gK (EK - V)"/1 -> Product/2

== system CurrentsLib/KAh_beta ==
  v : Inport
  Bias : Bias  Bias=1.2
  Gain : Gain  Gain=0
  s : Outport
  wires:
  Gain/1 -> Bias/1
  v/1 -> Gain/1
  Bias/1 -> s/1

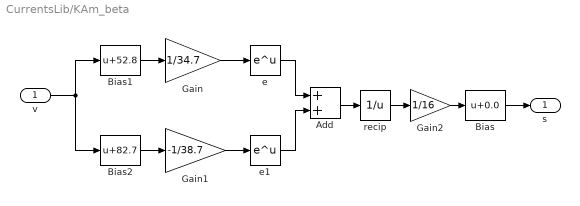
== system CurrentsLib/KAm_beta ==
  v : Inport
  Add : Sum
  Bias : Bias  Bias=0.0
  Bias1 : Bias  Bias=52.8
  Bias2 : Bias  Bias=82.7
  Gain : Gain  Gain=1/34.7
  Gain1 : Gain  Gain=-1/38.7
  Gain2 : Gain  Gain=1/16
  e : Math  SaturateOnIntegerOverflow=on
  e1 : Math  SaturateOnIntegerOverflow=on
  recip : Math  Operator=reciprocal  SaturateOnIntegerOverflow=on
  s : Outport
  wires:
  v/1 -> Bias1/1, Bias2/1
  Bias/1 -> s/1
  Bias2/1 -> Gain1/1
  Bias1/1 -> Gain/1
  Gain1/1 -> e1/1
  Gain/1 -> e/1
  e/1 -> Add/1
  e1/1 -> Add/2
  Add/1 -> recip/1
  Gain2/1 -> Bias/1
  recip/1 -> Gain2/1

== system CurrentsLib/L-type Ca Current , ICaL ==
  note: I_{CaL} = g_{CaL} m(V) p(V) Ighk
  V : Inport
  ca : Inport  Port=2
  GHK-I-Eq : CurrentsLib/GHK-I-Eq  SystemSampleTime=-1  z=2  Xi=10*10^(-6)  Xo=5  P=3.4*10^(-5)
  Gain : Gain  Gain=gCaL
  Product : Product  Inputs=3  RndMeth=Zero
  h Equil-Eqs Gate : Subsystem  mask{equilF=caLh_infin2, tauF=cah_tau2}
      mask prompts: equilF "Equilbrium Eq (Steady State)"; tauF "Tau Eq (Time constant)"
      mask help: dF/dt = ( infty_F-F) / tau_F
      mask init:
      | set_param([gcb '/TauFunct'], 'BlockChoice', tauF);
      | set_param([gcb '/EquilFunct'], 'BlockChoice', equilF);
      mask Help: dF/dt = ( infty_F-F) / tau_F
      mask StyleString: popup(caLm_infin|caLh_infin|caLm_infin2|caLh_infin2|caNm_infin2|caNh_infin2|caPm_infin2|caPh_infin2),popup(caLm_tau|caLh_tau|cam_tau2|cah_tau2)
      mask Display: image(imread('..\Libs\icons\EquilEq.jpg'),'center');
  m Equil-Eqs Gate : CurrentsLib/Equil-Eqs Gate  SystemSampleTime=-1  equilF=caLm_infin2  tauF=cam_tau2
  I : Outport
  wires:
  Product/1 -> I/1
  GHK-I-Eq/1 -> Gain/1
  V/1 -> h Equil-Eqs Gate/1(V), GHK-I-Eq/1, m Equil-Eqs Gate/1
  m Equil-Eqs Gate/1 -> Product/1
  h Equil-Eqs Gate/1(State) -> Product/2
  Gain/1 -> Product/3
  ca/1 -> GHK-I-Eq/2

== system CurrentsLib/M Current, IKM ==
  note: I_{K} = g_{K} m (E_{K} - V)
  V : Inport
  Product : Product  RndMeth=Zero
  "Ungated Current, gK (EK - V)" : CurrentsLib/Ungated Current  SystemSampleTime=-1  EX=EK  gX=gK
  m Rate-Eqs Gate : CurrentsLib/Rate-Eqs Gate  SystemSampleTime=-1  alphaF=kMm_alpha  betaF=kMm_beta
  I : Outport
  wires:
  "Ungated Current, gK (EK - V)"/1 -> Product/2
  Product/1 -> I/1
  m Rate-Eqs Gate/1 -> Product/1
  V/1 -> "Ungated Current, gK (EK - V)"/1, m Rate-Eqs Gate/1

== system CurrentsLib/N-type Ca Current, ICaN ==
  note: I_{CaN} = g_{CaN} m h (E_{CaN} - V)
  V : Inport
  ca : Inport  Port=2
  GHK-I-Eq : CurrentsLib/GHK-I-Eq  SystemSampleTime=-1  z=2  Xi=10*10^(-6)  Xo=5  P=3.4*10^(-5)
  Gain : Gain  Gain=gCaN
  Product : Product  Inputs=3  RndMeth=Zero
  h Equil Eqs Gate : Subsystem  mask{equilF=caNh_infin2, tauF=cah_tau2}
      mask prompts: equilF "Equilbrium Eq (Steady State)"; tauF "Tau Eq (Time constant)"
      mask help: dF/dt = ( infty_F-F) / tau_F
      mask init:
      | set_param([gcb '/TauFunct'], 'BlockChoice', tauF);
      | set_param([gcb '/EquilFunct'], 'BlockChoice', equilF);
      mask Help: dF/dt = ( infty_F-F) / tau_F
      mask StyleString: popup(caLm_infin|caLh_infin|caLm_infin2|caLh_infin2|caNm_infin2|caNh_infin2|caPm_infin2|caPh_infin2),popup(caLm_tau|caLh_tau|cam_tau2|cah_tau2)
      mask Display: image(imread('..\Libs\icons\EquilEq.jpg'),'center');
  m Equil Eqs Gate : CurrentsLib/Equil-Eqs Gate  SystemSampleTime=-1  equilF=caNm_infin2  tauF=cam_tau2
  I : Outport
  wires:
  h Equil Eqs Gate/1(State) -> Product/2
  m Equil Eqs Gate/1 -> Product/1
  V/1 -> m Equil Eqs Gate/1, h Equil Eqs Gate/1(V), GHK-I-Eq/1
  GHK-I-Eq/1 -> Gain/1
  Product/1 -> I/1
  Gain/1 -> Product/3
  ca/1 -> GHK-I-Eq/2

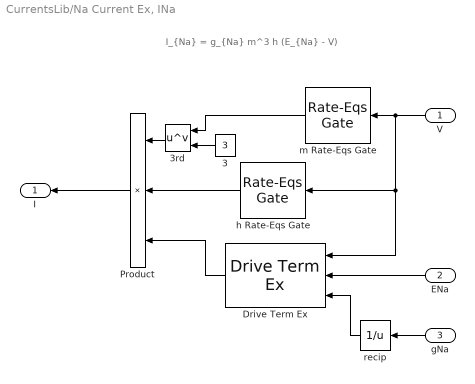
== system CurrentsLib/Na Current Ex, INa ==
  note: I_{Na} = g_{Na} m^3 h (E_{Na} - V)
  V : Inport
  ENa : Inport  Port=2
  gNa : Inport  Port=3
  " 3" : Constant  Value=3
  3rd : Math  Operator=pow  SaturateOnIntegerOverflow=on
  Drive Term Ex : WaveformsLib/Drive Term Ex  SystemSampleTime=-1
  Product : Product  Inputs=3  RndMeth=Zero
  h Rate-Eqs Gate : CurrentsLib/Rate-Eqs Gate  SystemSampleTime=-1  alphaF=h3_alpha  betaF=h3_beta
  m Rate-Eqs Gate : CurrentsLib/Rate-Eqs Gate  SystemSampleTime=-1  alphaF=m3_alpha  betaF=m3_beta
  recip : Math  Operator=reciprocal  SaturateOnIntegerOverflow=on
  I : Outport
  wires:
  Product/1 -> I/1
  V/1 -> m Rate-Eqs Gate/1, h Rate-Eqs Gate/1, Drive Term Ex/1
  " 3"/1 -> 3rd/2
  m Rate-Eqs Gate/1 -> 3rd/1
  3rd/1 -> Product/1
  h Rate-Eqs Gate/1 -> Product/2
  Drive Term Ex/1 -> Product/3
  ENa/1 -> Drive Term Ex/2
  gNa/1 -> recip/1
  recip/1 -> Drive Term Ex/3

== system CurrentsLib/Na Current, INa ==
  note: I_{Na} = g_{Na} m^3 h (E_{Na} - V)
  V : Inport
  " 3" : Constant  Value=3
  3rd : Math  Operator=pow  SaturateOnIntegerOverflow=on
  Product : Product  Inputs=3  RndMeth=Zero
  "Ungated Current, gNa (ENa - V)" : CurrentsLib/Ungated Current  SystemSampleTime=-1  EX=ENa  gX=gNa
  h Rate-Eqs Gate : CurrentsLib/Rate-Eqs Gate  SystemSampleTime=-1  alphaF=h3_alpha  betaF=h3_beta
  m Rate-Eqs Gate : CurrentsLib/Rate-Eqs Gate  SystemSampleTime=-1  alphaF=m3_alpha  betaF=m3_beta
  I : Outport
  wires:
  h Rate-Eqs Gate/1 -> Product/2
  3rd/1 -> Product/1
  m Rate-Eqs Gate/1 -> 3rd/1
  " 3"/1 -> 3rd/2
  V/1 -> m Rate-Eqs Gate/1, h Rate-Eqs Gate/1, "Ungated Current, gNa (ENa - V)"/1
  "Ungated Current, gNa (ENa - V)"/1 -> Product/3
  Product/1 -> I/1

== system CurrentsLib/P-type Ca Current, ICaP ==
  note: I_{CaN} = g_{CaN} m h (E_{CaN} - V)
  V : Inport
  ca : Inport  Port=2
  GHK-I-Eq : CurrentsLib/GHK-I-Eq  SystemSampleTime=-1  z=2  Xi=10*10^(-6)  Xo=5  P=3.4*10^(-5)
  Gain : Gain  Gain=gCaP
  Product : Product  Inputs=3  RndMeth=Zero
  h Equil-Eqs Gate : Subsystem  mask{equilF=caPh_infin2, tauF=cah_tau2}
      mask prompts: equilF "Equilbrium Eq (Steady State)"; tauF "Tau Eq (Time constant)"
      mask help: dF/dt = ( infty_F-F) / tau_F
      mask init:
      | set_param([gcb '/TauFunct'], 'BlockChoice', tauF);
      | set_param([gcb '/EquilFunct'], 'BlockChoice', equilF);
      mask Help: dF/dt = ( infty_F-F) / tau_F
      mask StyleString: popup(caLm_infin|caLh_infin|caLm_infin2|caLh_infin2|caNm_infin2|caNh_infin2|caPm_infin2|caPh_infin2),popup(caLm_tau|caLh_tau|cam_tau2|cah_tau2)
      mask Display: image(imread('..\Libs\icons\EquilEq.jpg'),'center');
  m EquilEqs Gate : CurrentsLib/Equil-Eqs Gate  SystemSampleTime=-1  equilF=caPm_infin2  tauF=cam_tau2
  I : Outport
  wires:
  Product/1 -> I/1
  Gain/1 -> Product/3
  V/1 -> m EquilEqs Gate/1, h Equil-Eqs Gate/1(V), GHK-I-Eq/1
  m EquilEqs Gate/1 -> Product/1
  h Equil-Eqs Gate/1(State) -> Product/2
  GHK-I-Eq/1 -> Gain/1
  ca/1 -> GHK-I-Eq/2

== system CurrentsLib/Rate- to Equil- Eq ==
  alpha : Inport
  beta : Inport  Port=2
  Add : Sum
  Math Function : Math  Operator=reciprocal  SaturateOnIntegerOverflow=on
  Product : Product  RndMeth=Zero
  infin : Outport
  tau : Outport  Port=2
  wires:
  alpha/1 -> Add/1, Product/1
  beta/1 -> Add/2
  Add/1 -> Math Function/1
  Product/1 -> infin/1
  Math Function/1 -> Product/2, tau/1

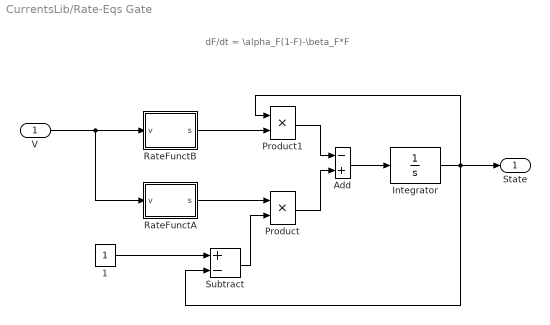
== system CurrentsLib/Rate-Eqs Gate ==
  note: dF/dt = \alpha_F(1-F)-\beta_F*F
  V : Inport
  1 : Constant
  Add : Sum  Inputs=-+
  Integrator : Integrator
  Product : Product  RndMeth=Zero
  Product1 : Product  RndMeth=Zero
  RateFunctA : Subsystem  BlockChoice=m3_alpha
      settings: AttributesFormatString=%<BlockChoice>  TemplateBlock=CurrentsLib/RateFunct  MemberBlocks=KAh_alpha,KAh_beta,KAm_alpha,KAm_beta,caLh_infin,caLh_infin2,caLh_tau,caLm_infin,caLm_infin2,caLm_tau,caNh_infin2,caNm_infin2,caPh_infin2,caPm_infin2,cah_tau2,cam_tau2,h2_alpha,h2_beta,h3_alpha,h3_beta,h4_alpha,h4_beta,h_alpha,h_beta,kMm_alpha,kMm_beta,m2_alpha,m2_beta,m3_alpha,m3_beta,m4_alpha,m4_beta,m_alpha,m_beta,n2_alpha,n2_beta,n3_alpha,n3_beta,n4_alpha,n4_beta,n_alpha,n_beta
  RateFunctB : Subsystem  BlockChoice=m3_beta
      settings: AttributesFormatString=%<BlockChoice>  TemplateBlock=CurrentsLib/RateFunct  MemberBlocks=KAh_alpha,KAh_beta,KAm_alpha,KAm_beta,caLh_infin,caLh_infin2,caLh_tau,caLm_infin,caLm_infin2,caLm_tau,caNh_infin2,caNm_infin2,caPh_infin2,caPm_infin2,cah_tau2,cam_tau2,h2_alpha,h2_beta,h3_alpha,h3_beta,h4_alpha,h4_beta,h_alpha,h_beta,kMm_alpha,kMm_beta,m2_alpha,m2_beta,m3_alpha,m3_beta,m4_alpha,m4_beta,m_alpha,m_beta,n2_alpha,n2_beta,n3_alpha,n3_beta,n4_alpha,n4_beta,n_alpha,n_beta
  Subtract : Sum  Inputs=+-
  State : Outport
  wires:
  RateFunctB/1(s) -> Product1/2
  Product1/1 -> Add/1
  RateFunctA/1(s) -> Product/1
  V/1 -> RateFunctB/1(v), RateFunctA/1(v)
  Product/1 -> Add/2
  Subtract/1 -> Product/2
  1/1 -> Subtract/1
  Integrator/1 -> Product1/1, State/1, Subtract/2
  Add/1 -> Integrator/1

== system CurrentsLib/RateFunct ==
  v : Inport
  m_alpha : CurrentsLib/StateFunctFormI  SystemSampleTime=-1  T=-47  S=1/4  M=-1  B=1  G=0.32
  s : Outport
  wires:
  v/1 -> m_alpha/1
  m_alpha/1 -> s/1

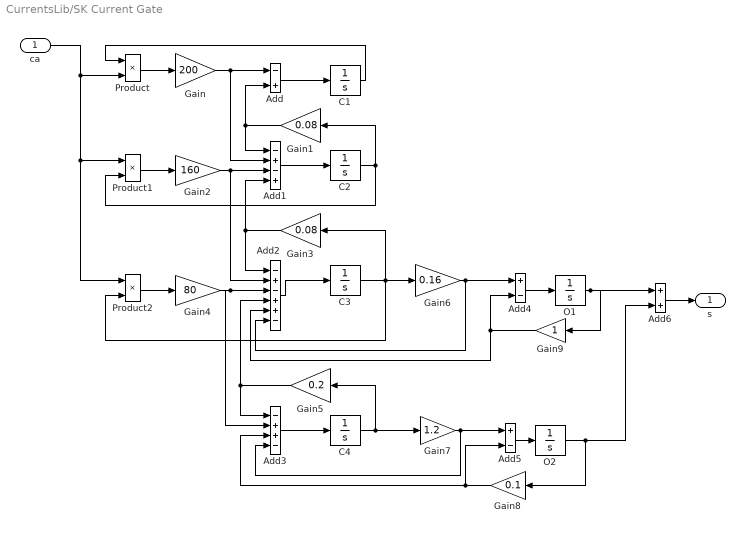
== system CurrentsLib/SK Current Gate ==
  ca : Inport
  Add : Sum  Inputs=-+
  Add1 : Sum  Inputs=-+-+
  Add2 : Sum  Inputs=-+-++-
  Add3 : Sum  Inputs=-++-
  Add4 : Sum  Inputs=+-
  Add5 : Sum  Inputs=+-
  Add6 : Sum
  C1 : Integrator  InitialCondition=1
  C2 : Integrator
  C3 : Integrator
  C4 : Integrator
  Gain : Gain  Gain=200
  Gain1 : Gain  Gain=0.08
  Gain2 : Gain  Gain=160
  Gain3 : Gain  Gain=0.08
  Gain4 : Gain  Gain=80
  Gain5 : Gain  Gain=0.2
  Gain6 : Gain  Gain=0.16
  Gain7 : Gain  Gain=1.2
  Gain8 : Gain  Gain=0.1
  Gain9 : Gain
  O1 : Integrator
  O2 : Integrator
  Product : Product  RndMeth=Zero
  Product1 : Product  RndMeth=Zero
  Product2 : Product  RndMeth=Zero
  s : Outport
  wires:
  C1/1 -> Product/1
  ca/1 -> Product/2, Product1/1, Product2/1
  Product/1 -> Gain/1
  Gain/1 -> Add/1, Add1/2
  Add/1 -> C1/1
  C2/1 -> Gain1/1, Product1/2
  Gain1/1 -> Add/2, Add1/1
  Product1/1 -> Gain2/1
  Gain2/1 -> Add1/3, Add2/2
  C3/1 -> Gain3/1, Product2/2, Gain6/1
  Gain3/1 -> Add1/4, Add2/1
  Add1/1 -> C2/1
  Add2/1 -> C3/1
  Product2/1 -> Gain4/1
  Gain4/1 -> Add2/3, Add3/2
  C4/1 -> Gain5/1, Gain7/1
  Gain5/1 -> Add2/4, Add3/1
  Add5/1 -> O2/1
  Add4/1 -> O1/1
  O1/1 -> Add6/1, Gain9/1
  Gain6/1 -> Add2/6, Add4/1
  O2/1 -> Gain8/1, Add6/2
  Gain8/1 -> Add5/2, Add3/3
  Add3/1 -> C4/1
  Gain7/1 -> Add5/1, Add3/4
  Add6/1 -> s/1
  Gain9/1 -> Add2/5, Add4/2

== system CurrentsLib/Seq Gate ==
  note: dF/dt = in-out*F
  in : Inport
  out : Inport  Port=2
  Add : Sum  Inputs=+-
  Integrator : Integrator  InitialCondition=S0
  Product1 : Product  RndMeth=Zero
  State : Outport
  wires:
  Add/1 -> Integrator/1
  Integrator/1 -> State/1, Product1/2
  out/1 -> Product1/1
  in/1 -> Add/1
  Product1/1 -> Add/2

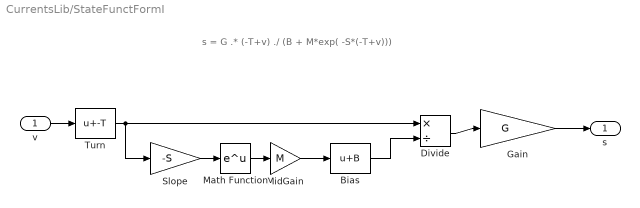
== system CurrentsLib/StateFunctFormI ==
  note: s = G .* (-T+v) ./ (B + M*exp( -S*(-T+v)))
  v : Inport
  Bias : Bias  Bias=B
  Divide : Product  Inputs=*/
  Gain : Gain  Gain=G
  Math Function : Math  SaturateOnIntegerOverflow=on
  MidGain : Gain  Gain=M
  Slope : Gain  Gain=-S
  Turn : Bias  Bias=-T
  s : Outport
  wires:
  Turn/1 -> Divide/1, Slope/1
  Slope/1 -> Math Function/1
  Math Function/1 -> MidGain/1
  Bias/1 -> Divide/2
  Divide/1 -> Gain/1
  v/1 -> Turn/1
  Gain/1 -> s/1
  MidGain/1 -> Bias/1

== system CurrentsLib/StateFunctFormII ==
  note: s = G .* exp( -S*(-T+v)))
  v : Inport
  Gain : Gain  Gain=G
  Math Function : Math  SaturateOnIntegerOverflow=on
  Slope : Gain  Gain=-S
  Turn : Bias  Bias=-T
  s : Outport
  wires:
  Turn/1 -> Slope/1
  Slope/1 -> Math Function/1
  v/1 -> Turn/1
  Gain/1 -> s/1
  Math Function/1 -> Gain/1

== system CurrentsLib/StateFunctFormIII ==
  note: s = G ./ (exp( -S*(-T+v)) + B)
  v : Inport
  Gain : Gain  Gain=G
  Slope : Gain  Gain=-S
  Turn : Bias  Bias=-T
  Turn1 : Bias  Bias=B
  exp : Math  SaturateOnIntegerOverflow=on
  recip : Math  Operator=reciprocal  SaturateOnIntegerOverflow=on
  s : Outport
  wires:
  exp/1 -> Turn1/1
  Gain/1 -> s/1
  v/1 -> Turn/1
  Slope/1 -> exp/1
  Turn/1 -> Slope/1
  Turn1/1 -> recip/1
  recip/1 -> Gain/1

== system CurrentsLib/TauFunct ==
  v : Inport
  caLh_tau : CurrentsLib/caLh_tau  SystemSampleTime=-1
  s : Outport
  wires:
  v/1 -> caLh_tau/1
  caLh_tau/1 -> s/1

== system CurrentsLib/Ungated Current ==
  note: I_{X} = g_{X} (E_{X} - V)
  V : Inport
  Drive Term : WaveformsLib/Drive Term  SystemSampleTime=-1  EX=EX  tauX=1/gX
  I : Outport
  wires:
  Drive Term/1 -> I/1
  V/1 -> Drive Term/1

== system CurrentsLib/V-gated sAHP, IvsAHP ==
  spike : Inport
  v : Inport  Port=2
  Product : Product  RndMeth=Zero
  Ungated Current : CurrentsLib/Ungated Current  SystemSampleTime=-1  EX=EvsAHP  gX=gvsAHP
  sAHP Compound Diff : WaveformsLib/Compound Diffentials  SystemSampleTime=-1  tauRise=RvsAHP  tauFall=FvsAHP  squareWaveWidth=1  squareWaveHeight=1  interGain=4/RvsAHP  finalGain=1
  I : Outport
  wires:
  spike/1 -> sAHP Compound Diff/1
  Product/1 -> I/1
  v/1 -> Ungated Current/1
  Ungated Current/1 -> Product/2
  sAHP Compound Diff/2 -> Product/1

== system CurrentsLib/caLh_tau ==
  v : Inport
  Bias : Bias  Bias=420
  Gain : Gain  Gain=0
  s : Outport
  wires:
  Bias/1 -> s/1
  v/1 -> Gain/1
  Gain/1 -> Bias/1

== system CurrentsLib/caLm_tau ==
  v : Inport
  Bias : Bias  Bias=37.1
  Gain : Gain  Gain=1.25
  Gain1 : Gain  Gain=-0.031
  cosh : Trigonometry  Operator=cosh
  recip : Math  Operator=reciprocal  SaturateOnIntegerOverflow=on
  s : Outport
  wires:
  Gain/1 -> s/1
  v/1 -> Bias/1
  Bias/1 -> Gain1/1
  recip/1 -> Gain/1
  cosh/1 -> recip/1
  Gain1/1 -> cosh/1

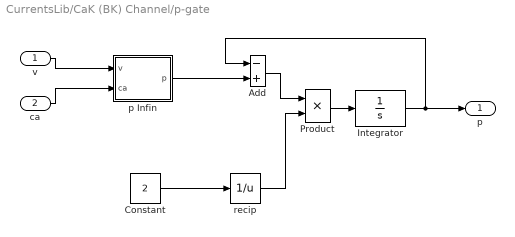
== system CurrentsLib/CaK (BK) Channel/p-gate ==
  v : Inport
  ca : Inport  Port=2
  Add : Sum  Inputs=-+
  Constant : Constant  Value=2
  Integrator : Integrator
  Product : Product  RndMeth=Zero
  p Infin : Subsystem
  recip : Math  Operator=reciprocal  SaturateOnIntegerOverflow=on
  p : Outport
  wires:
  Constant/1 -> recip/1
  Integrator/1 -> p/1, Add/1
  Add/1 -> Product/1
  Product/1 -> Integrator/1
  recip/1 -> Product/2
  v/1 -> p Infin/1(v)
  p Infin/1(p) -> Add/2
  ca/1 -> p Infin/2(ca)

== system CurrentsLib/Equil-Eqs Gate/EquilFunct ==
  v : Inport
  caLh_infin : CurrentsLib/StateFunctFormIII  SystemSampleTime=-1  T=-12.6  S=1/18.9  B=1  G=1
  s : Outport
  wires:
  v/1 -> caLh_infin/1
  caLh_infin/1 -> s/1

== system CurrentsLib/Equil-Eqs Gate/TauFunct ==
  v : Inport
  caLh_tau : CurrentsLib/caLh_tau  SystemSampleTime=-1
  s : Outport
  wires:
  v/1 -> caLh_tau/1
  caLh_tau/1 -> s/1

== system CurrentsLib/L-type Ca Current , ICaL/h Equil-Eqs Gate ==
  note: dF/dt = ( \infty _F-F) / \tau_F
  V : Inport
  Add1 : Sum  Inputs=-+
  Divide : Product  Inputs=*/
  EquilFunct : Subsystem  BlockChoice=caLh_infin2
      settings: AttributesFormatString=%<BlockChoice>  TemplateBlock=CurrentsLib/EquilFunct  MemberBlocks=caLh_infin,caLh_infin2,caLm_infin,caLm_infin2,caNh_infin2,caNm_infin2,caPh_infin2,caPm_infin2
  Integrator : Integrator  InitialCondition=1
  TauFunct : Subsystem  BlockChoice=cah_tau2
      settings: AttributesFormatString=%<BlockChoice>  TemplateBlock=CurrentsLib/TauFunct  MemberBlocks=caLh_tau,caLm_tau,cah_tau2,cam_tau2
  State : Outport
  wires:
  V/1 -> EquilFunct/1(v), TauFunct/1(v)
  EquilFunct/1(s) -> Add1/2
  TauFunct/1(s) -> Divide/2
  Divide/1 -> Integrator/1
  Add1/1 -> Divide/1
  Integrator/1 -> State/1, Add1/1

== system CurrentsLib/N-type Ca Current, ICaN/h Equil Eqs Gate ==
  note: dF/dt = ( \infty _F-F) / \tau_F
  V : Inport
  Add1 : Sum  Inputs=-+
  Divide : Product  Inputs=*/
  EquilFunct : Subsystem  BlockChoice=caNh_infin2
      settings: AttributesFormatString=%<BlockChoice>  TemplateBlock=CurrentsLib/EquilFunct  MemberBlocks=caLh_infin,caLh_infin2,caLm_infin,caLm_infin2,caNh_infin2,caNm_infin2,caPh_infin2,caPm_infin2
  Integrator : Integrator  InitialCondition=1
  TauFunct : Subsystem  BlockChoice=cah_tau2
      settings: AttributesFormatString=%<BlockChoice>  TemplateBlock=CurrentsLib/TauFunct  MemberBlocks=caLh_tau,caLm_tau,cah_tau2,cam_tau2
  State : Outport
  wires:
  V/1 -> EquilFunct/1(v), TauFunct/1(v)
  EquilFunct/1(s) -> Add1/2
  TauFunct/1(s) -> Divide/2
  Divide/1 -> Integrator/1
  Add1/1 -> Divide/1
  Integrator/1 -> State/1, Add1/1

== system CurrentsLib/P-type Ca Current, ICaP/h Equil-Eqs Gate ==
  note: dF/dt = ( \infty _F-F) / \tau_F
  V : Inport
  Add1 : Sum  Inputs=-+
  Divide : Product  Inputs=*/
  EquilFunct : Subsystem  BlockChoice=caPh_infin2
      settings: AttributesFormatString=%<BlockChoice>  TemplateBlock=CurrentsLib/EquilFunct  MemberBlocks=caLh_infin,caLh_infin2,caLm_infin,caLm_infin2,caNh_infin2,caNm_infin2,caPh_infin2,caPm_infin2
  Integrator : Integrator  InitialCondition=1
  TauFunct : Subsystem  BlockChoice=cah_tau2
      settings: AttributesFormatString=%<BlockChoice>  TemplateBlock=CurrentsLib/TauFunct  MemberBlocks=caLh_tau,caLm_tau,cah_tau2,cam_tau2
  State : Outport
  wires:
  V/1 -> EquilFunct/1(v), TauFunct/1(v)
  EquilFunct/1(s) -> Add1/2
  TauFunct/1(s) -> Divide/2
  Divide/1 -> Integrator/1
  Add1/1 -> Divide/1
  Integrator/1 -> State/1, Add1/1

== system CurrentsLib/Rate-Eqs Gate/RateFunctA ==
  v : Inport
  m3_alpha : CurrentsLib/StateFunctFormI  SystemSampleTime=-1  T=-47  S=0.25  M=-1  B=1  G=0.32
  s : Outport
  wires:
  v/1 -> m3_alpha/1
  m3_alpha/1 -> s/1

== system CurrentsLib/Rate-Eqs Gate/RateFunctB ==
  v : Inport
  m3_beta : CurrentsLib/StateFunctFormI  SystemSampleTime=-1  T=-20  S=-0.2  M=1  B=-1  G=0.28
  s : Outport
  wires:
  v/1 -> m3_beta/1
  m3_beta/1 -> s/1

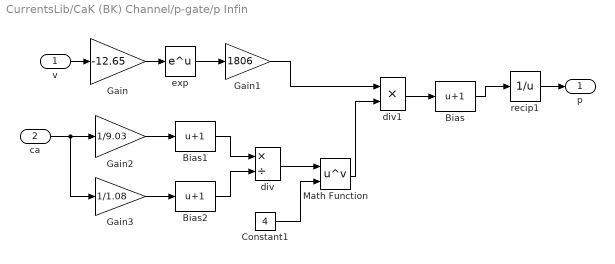
== system CurrentsLib/CaK (BK) Channel/p-gate/p Infin ==
  v : Inport
  ca : Inport  Port=2
  Bias : Bias  Bias=1
  Bias1 : Bias  Bias=1
  Bias2 : Bias  Bias=1
  Constant1 : Constant  Value=4
  Gain : Gain  Gain=-12.65
  Gain1 : Gain  Gain=1806
  Gain2 : Gain  Gain=1/9.03
  Gain3 : Gain  Gain=1/1.08
  Math Function : Math  Operator=pow  SaturateOnIntegerOverflow=on
  div : Product  Inputs=*/  RndMeth=Zero
  div1 : Product  RndMeth=Zero
  exp : Math  SaturateOnIntegerOverflow=on
  recip1 : Math  Operator=reciprocal  SaturateOnIntegerOverflow=on
  p : Outport
  wires:
  Gain/1 -> exp/1
  exp/1 -> Gain1/1
  ca/1 -> Gain2/1, Gain3/1
  Gain2/1 -> Bias1/1
  Gain3/1 -> Bias2/1
  Bias1/1 -> div/1
  Bias2/1 -> div/2
  div/1 -> Math Function/1
  Constant1/1 -> Math Function/2
  Gain1/1 -> div1/1
  Math Function/1 -> div1/2
  div1/1 -> Bias/1
  Bias/1 -> recip1/1
  v/1 -> Gain/1
  recip1/1 -> p/1
